simulink model "suspension_sys_Simulink"  (Simulink 9.1)
settings: Solver=ode45  StartTime=0.0  StopTime=10.0  RelTol=1e-3  EnableMultiTasking=on
model workspace (MAT data in the model file):
  Ks = 28000
  Kse = 8000
  Kt = 125000
  M1 = 2500
  M2 = 320
  Ms = 250
  Mse = 90
  Mu = 40
  Zr = 0.2
  b1 = 350
  b2 = 15020
  bs = 2000
  bse = 3000
  k1 = 80000
  k2 : num (value not decoded)
values from neighbouring files (symbols this model uses):
  bs = 2000    [suspensiondata.mat]
  bse = 3000    [suspensiondata.mat]
  Kse = 8000    [suspensiondata.mat]
  Kt = 125000    [suspensiondata.mat]
  Ms = 250    [suspensiondata.mat]
  Mse = 90    [suspensiondata.mat]
  Mu = 40    [suspensiondata.mat]
settings Model: Creator=kiran.jacob  LastModifiedBy=Saurabh Suman
settings DataIOCC: LimitDataPoints=on  SignalLoggingSaveFormat=ModelDataLogs
settings OptimizationCC: ExpressionDepthLimit=2147483647  InitFltsAndDblsToZero=on
settings DebuggingCC: SolverPrmCheckMsg=warning  FcnCallInpInsideContextMsg=warning  StateNameClashWarn=warning

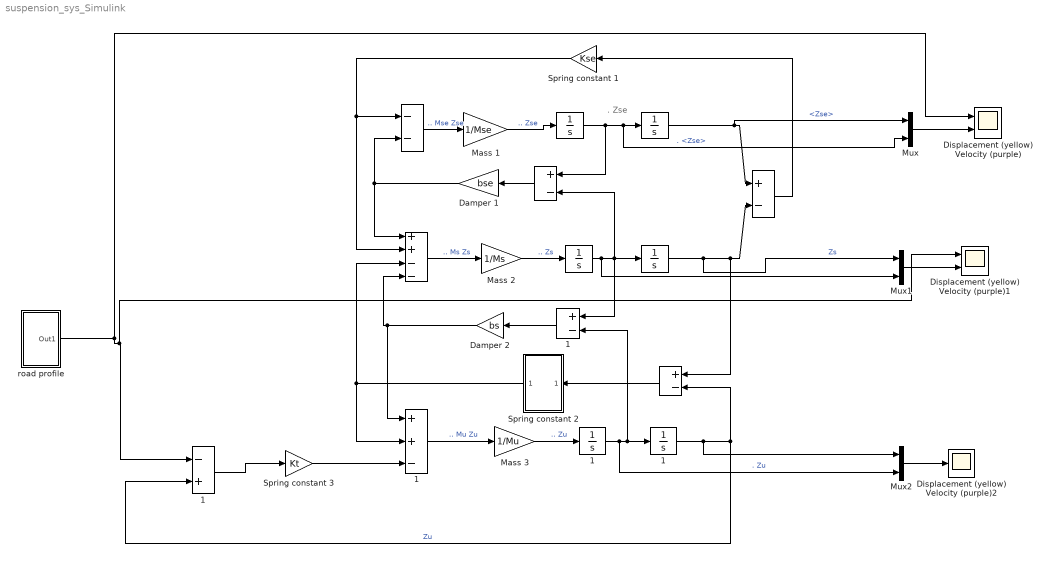
== system suspension_sys_Simulink ==
  note: .
      | Zse
  " " : Integrator
  "  " : Sum  Inputs=+-
  "     " : Integrator
  "      " : Sum  Inputs=++--
  "       " : Sum  Inputs=--
  "        " : Sum  Inputs=+-
  "         " : Integrator
  "          " : Integrator
  "             " : Sum  Inputs=+-
  "             1" : Sum  Inputs=+-
  "          1" : Integrator
  "         1" : Integrator
  "       1" : Sum  Inputs=-+
  "      1" : Sum  Inputs=++-
  Damper 1 : Gain  Gain=bse
  Damper 2 : Gain  Gain=bs
  Displacement (yellow) Velocity (purple) : Scope  NumInputPorts=2
  Displacement (yellow) Velocity (purple)1 : Scope  NumInputPorts=2
  Displacement (yellow) Velocity (purple)2 : Scope
  Mass 1 : Gain  Gain=1/Mse
  Mass 2 : Gain  Gain=1/Ms
  Mass 3 : Gain  Gain=1/Mu
  Mux : Mux  Inputs=2
  Mux1 : Mux  Inputs=2
  Mux2 : Mux  Inputs=2
  Spring constant 1 : Gain  Gain=Kse
  Spring constant 2 : Subsystem
  Spring constant 3 : Gain  Gain=Kt
  road profile : Subsystem
  wires:
  " "/1 -> "        "/1, "     "/1, Mux/2  ". <Zse>"
  "         "/1 -> "        "/2, "          "/1, "             1"/1, Mux1/2
  Mass 1/1 -> " "/1  ".. Zse"
  Mass 2/1 -> "         "/1  ".. Zs"
  "       "/1 -> Mass 1/1  ".. Mse Zse"
  "      "/1 -> Mass 2/1  ".. Ms Zs"
  "     "/1 -> "  "/1, Mux/1  "<Zse>"
  "          "/1 -> "  "/2, "             "/1, Mux1/1  "Zs"
  "  "/1 -> Spring constant 1/1
  Spring constant 1/1 -> "      "/2, "       "/1
  "        "/1 -> Damper 1/1
  Damper 1/1 -> "      "/1, "       "/2
  "      1"/1 -> Mass 3/1  ".. Mu Zu"
  Mass 3/1 -> "         1"/1  ".. Zu"
  "         1"/1 -> "          1"/1, "             1"/2, Mux2/2  ". Zu"
  "          1"/1 -> "             "/2, "       1"/2, Mux2/1  "Zu"
  "             "/1 -> Spring constant 2/1(In3)
  "             1"/1 -> Damper 2/1
  Damper 2/1 -> "      "/4, "      1"/1
  Spring constant 2/1(Out1) -> "      "/3, "      1"/2
  Spring constant 3/1 -> "      1"/3
  "       1"/1 -> Spring constant 3/1
  Mux2/1 -> Displacement (yellow) Velocity (purple)2/1
  Mux/1 -> Displacement (yellow) Velocity (purple)/2
  Mux1/1 -> Displacement (yellow) Velocity (purple)1/2
  road profile/1(Out1) -> Displacement (yellow) Velocity (purple)/1, Displacement (yellow) Velocity (purple)1/1, "       1"/1

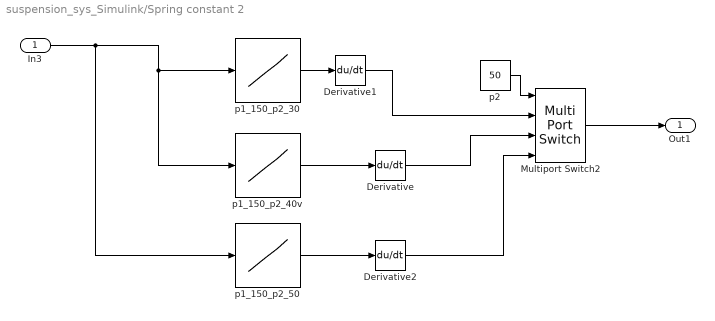
== system suspension_sys_Simulink/Spring constant 2 ==
  In3 : Inport
  Derivative : Derivative
  Derivative1 : Derivative
  Derivative2 : Derivative
  Multiport Switch2 : MultiPortSwitch  DataPortOrder=Specify indices  DataPortIndices={30,40,50}
  p1_150_p2_30 : Lookup_n-D  NumberOfTableDimensions=1  BreakpointsForDimension1=p1_150_p2_30v(1:end,1)  Table=p1_150_p2_30v(1:end,2)  TableDataTypeStr=Inherit: Inherit from 'Table data'  DiagnosticForOutOfRangeInput=Warning  InternalRulePriority=Speed  RndMeth=Simplest  InputSameDT=on
  p1_150_p2_40v : Lookup_n-D  NumberOfTableDimensions=1  BreakpointsForDimension1=p1_150_p2_40v(1:end,1)  Table=p1_150_p2_40v(1:end,2)  TableDataTypeStr=Inherit: Inherit from 'Table data'  InternalRulePriority=Speed  RndMeth=Simplest  InputSameDT=on
  p1_150_p2_50 : Lookup_n-D  NumberOfTableDimensions=1  BreakpointsForDimension1=p1_150_p2_50v(1:end,1)  Table=p1_150_p2_50v(1:end,2)  TableDataTypeStr=Inherit: Inherit from 'Table data'  InternalRulePriority=Speed  RndMeth=Simplest  InputSameDT=on
  p2 : Constant  Value=50
  Out1 : Outport
  wires:
  Multiport Switch2/1 -> Out1/1
  p1_150_p2_40v/1 -> Derivative/1
  p2/1 -> Multiport Switch2/1
  In3/1 -> p1_150_p2_50/1, p1_150_p2_30/1, p1_150_p2_40v/1
  p1_150_p2_50/1 -> Derivative2/1
  p1_150_p2_30/1 -> Derivative1/1
  Derivative/1 -> Multiport Switch2/3
  Derivative2/1 -> Multiport Switch2/4
  Derivative1/1 -> Multiport Switch2/2

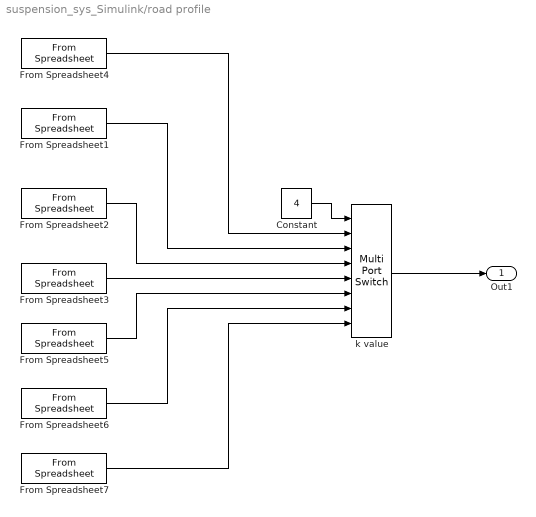
== system suspension_sys_Simulink/road profile ==
  Constant : Constant  Value=4
  From Spreadsheet1 : FromSpreadsheet  FileName=D:\Full vehicle MATLAB suspension model\road.xlsx  SheetName=k=4
  From Spreadsheet2 : FromSpreadsheet  FileName=D:\Full vehicle MATLAB suspension model\road.xlsx  SheetName=k=5
  From Spreadsheet3 : FromSpreadsheet  FileName=D:\Full vehicle MATLAB suspension model\road.xlsx  SheetName=k=6
  From Spreadsheet4 : FromSpreadsheet  FileName=D:\Full vehicle MATLAB suspension model\road.xlsx  SheetName=k=3
  From Spreadsheet5 : FromSpreadsheet  FileName=D:\Full vehicle MATLAB suspension model\road.xlsx  SheetName=k=3
  From Spreadsheet6 : FromSpreadsheet  FileName=D:\Full vehicle MATLAB suspension model\road.xlsx  SheetName=k=8
  From Spreadsheet7 : FromSpreadsheet  FileName=D:\Full vehicle MATLAB suspension model\road.xlsx  SheetName=k=9
  k value : MultiPortSwitch  DataPortOrder=Specify indices  Inputs=7  DataPortIndices={3,4,5,6,7,8,9}
  Out1 : Outport
  wires:
  From Spreadsheet2/1 -> k value/4
  From Spreadsheet5/1 -> k value/6
  From Spreadsheet1/1 -> k value/3
  From Spreadsheet4/1 -> k value/2
  From Spreadsheet6/1 -> k value/7
  Constant/1 -> k value/1
  From Spreadsheet7/1 -> k value/8
  From Spreadsheet3/1 -> k value/5
  k value/1 -> Out1/1
